simulink model "sistem"  (R2021a)
settings: Solver=VariableStepAuto  StartTime=0.0  StopTime=50.0  RelTol=1e-3
settings Model: Creator=Batikan  LastModifiedBy=Batikan

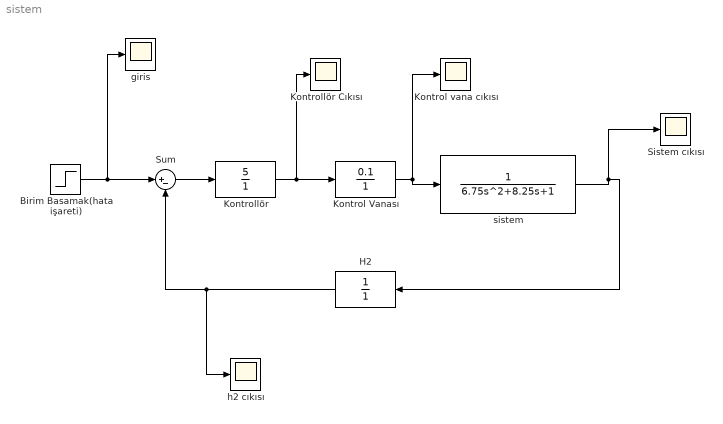
== system sistem ==
  " H2" : TransferFcn  Denominator=[1]
  Birim Basamak(hata işareti) : Step  SampleTime=0
  Kontrol Vanası : TransferFcn  Numerator=[0.1]  Denominator=[0 1]
  Kontrol vana cıkısı : Scope
  Kontrollör : TransferFcn  Numerator=[5]  Denominator=[0 1]
  Kontrollör Cıkısı : Scope
  Sistem cıkısı : Scope
  Sum : Sum  Inputs=|+-
  giris : Scope
  h2 cıkısı : Scope
  sistem : TransferFcn  Denominator=[6.75 8.25 1]
  wires:
  Birim Basamak(hata işareti)/1 -> giris/1, Sum/1
  Sum/1 -> Kontrollör/1
  " H2"/1 -> h2 cıkısı/1, Sum/2
  Kontrollör/1 -> Kontrollör Cıkısı/1, Kontrol Vanası/1
  Kontrol Vanası/1 -> Kontrol vana cıkısı/1, sistem/1
  sistem/1 -> Sistem cıkısı/1, " H2"/1
